simulink model "tank_non_linear_model"  (R2019b)
settings: Solver=VariableStepAuto  StartTime=0.0  StopTime=10.0  RelTol=1e-3
values from neighbouring files (symbols this model uses):
  Ts = 0.5    [workspace.mat]
  ue = [ue1; ue2]    [equibrium.m]    (also in equibrium.mat = [1.87816229294 0]; workspace.mat = [1.87816229294 0])
  xe = [xe1; xe2]    [equibrium.m]    (also in equibrium.mat = [24.8812336392 25.53]; workspace.mat = [24.8812336392 25.53])
settings Model: Creator=tongk  LastModifiedBy=tongk

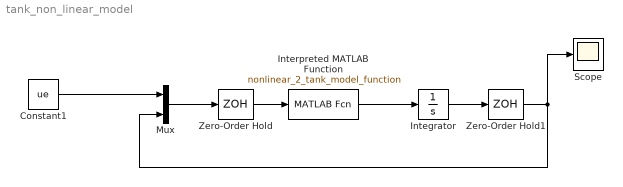
== system tank_non_linear_model ==
  Constant1 : Constant  Value=ue
  Integrator : Integrator  InitialCondition=xe
  Interpreted MATLAB Function : MATLABFcn  MATLABFcn=nonlinear_2_tank_model_function
  Mux : Mux  Inputs=2
  Scope : Scope
  Zero-Order Hold : ZeroOrderHold  SampleTime=Ts
  Zero-Order Hold1 : ZeroOrderHold  SampleTime=Ts
  wires:
  Zero-Order Hold/1 -> Interpreted MATLAB Function/1
  Zero-Order Hold1/1 -> Mux/2, Scope/1
  Interpreted MATLAB Function/1 -> Integrator/1
  Integrator/1 -> Zero-Order Hold1/1
  Mux/1 -> Zero-Order Hold/1
  Constant1/1 -> Mux/1
